simulink model "k1vissr3ta"  (Simulink 8.6)
settings: Solver=VariableStepAuto  StartTime=0.0  StopTime=10.0  RelTol=1e-3
libraries: cdsFilt x4, cdsCDO64 x3, cdsIPCx x3, TYPEB_MASTER x3, cdsCDI64 x2, dac x2, cdsAdcx0 x1, cdsParameters x1
settings Model: Creator=controls  LastModifiedBy=controls
settings DataIOCC: SaveFormat=Dataset  SignalLoggingSaveFormat=Dataset
settings OptimizationCC: ExpressionDepthLimit=128
settings DebuggingCC: UnderspecifiedInitializationDetection=Simplified  MergeDetectMultiDrivingBlocksExec=error  SolverPrmCheckMsg=none  FcnCallInpInsideContextMsg=EnableAllAsError  StateNameClashWarn=none
settings HardwareCC: ProdBitPerPointer=64  ProdLargestAtomicFloat=Float  ProdIntDivRoundTo=Zero  ProdEndianess=LittleEndian  ProdWordSize=64  ProdHWDeviceType=Intel->x86-64 (Windows64)
settings GRTTargetCC: GeneratePreprocessorConditionals=Use local settings  CombineOutputUpdateFcns=on  GRTInterface=off
settings ConfigComp: CovModelRefEnable=off

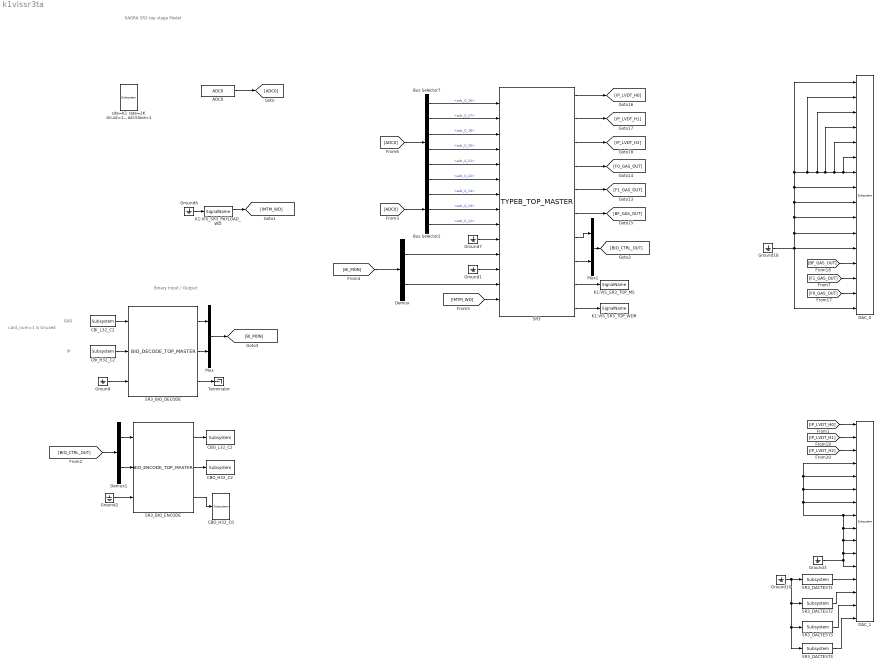
== system k1vissr3ta ==
  note: KAGRA SR3 top stage Model
  note: Binary Input / Output
  note: card_num=1 is Unused
  note: GAS
  note: IP
  ADC0 : cdsAdcx0/ADC0  Tag=cdsAdc  Description=|
      | type-GSC_16AI64SSA
      | card_num=0
      settings: AttributesFormatString=%<Description>\n%<Tag>
  Bus Selector2 : BusSelector  Description=ADC Selector  OutputSignals=adc_0_14,adc_0_13,adc_0_12
      settings: AttributesFormatString=%<Description>
  Bus Selector7 : BusSelector  Description=ADC Selector  OutputSignals=adc_0_16,adc_0_17,adc_0_18,adc_0_20,adc_0_21,adc_0_22
      settings: AttributesFormatString=%<Description>
  CBI_H32_C2 : cdsCDI64/Subsystem  Tag=cdsCDI64  Description=card_num=5
      settings: AttributesFormatString=%<Tag>\n%<Description>
  CBI_L32_C2 : cdsCDI64/Subsystem  Tag=cdsCDI64  Description=card_num=4
      settings: AttributesFormatString=%<Tag>\n%<Description>
  CBO_H32_C0 : cdsCDO64/Subsystem  Tag=cdsCDO64  Description=card_num=1
      settings: AttributesFormatString=%<Tag>\n%<Description>
  CBO_H32_C2 : cdsCDO64/Subsystem  Tag=cdsCDO64  Description=card_num=5
      settings: AttributesFormatString=%<Tag>\n%<Description>
  CBO_L32_C2 : cdsCDO64/Subsystem  Tag=cdsCDO64  Description=card_num=4
      settings: AttributesFormatString=%<Tag>\n%<Description>
  DAC_0 : dac/Subsystem  Description=|
      | type=GSC_16AO16,
      | card_num=0
      settings: AttributesFormatString=%<Description>
  DAC_1 : dac/Subsystem  Description=|
      | type=GSC_16AO16,
      | card_num=1
      settings: AttributesFormatString=%<Description>
  Demux : Demux  Outputs=2
  Demux1 : Demux  Outputs=2
  Ground{,1..3,6..7,10,18} (8 alike) : Ground
  K1:VIS_SR3_PAYLOAD_WD : cdsIPCx/SignalName  Tag=cdsIPCx_SHMEM  Description=Inter-Process Communication via Shared memory.
      settings: AttributesFormatString=%<Tag>
  K1:VIS_SR3_TOP_MS : cdsIPCx/SignalName  Tag=cdsIPCx_SHMEM  Description=Inter-Process Communication via Shared memory.
      settings: AttributesFormatString=%<Tag>
  K1:VIS_SR3_TOP_WDR : cdsIPCx/SignalName  Tag=cdsIPCx_SHMEM  Description=Inter-Process Communication via Shared memory.
      settings: AttributesFormatString=%<Tag>
  Mux : Mux  Inputs=2
  Mux1 : Mux  Inputs=2
  SR3 : TYPEB_MASTER/TYPEB_TOP_MASTER
  SR3_BIO_DECODE : TYPEB_MASTER/BIO_DECODE_TOP_MASTER
  SR3_BIO_ENCODE : TYPEB_MASTER/BIO_ENCODE_TOP_MASTER
  SR3_DACTEST1 : cdsFilt/Subsystem  Tag=cdsFilt  Description=|
      | Purpose:                                                                                                                                                                                                                                  
      | Standard CDS IIR filter module.                                                                                                                                                                                                           
      |                                                                                                                                                                                                                                           
      | Operation:                                                                                                                                                                                                                                
      | Consists of 10 second order section IIR filters, plus a ramped gain stage. In FE code, also provides pre-defined test points and excitation channel inputs. The filter coefficients are defined in the LIGO system using the 'foton' tool.
      |                                                                                                                                                                                                                                           
      | Usage:                                                                                                                                                                                                                                    
      | Name the part with the desired filter module name.
      settings: AttributesFormatString=%<Tag>
  SR3_DACTEST2 : cdsFilt/Subsystem  Tag=cdsFilt  Description=|
      | Purpose:                                                                                                                                                                                                                                  
      | Standard CDS IIR filter module.                                                                                                                                                                                                           
      |                                                                                                                                                                                                                                           
      | Operation:                                                                                                                                                                                                                                
      | Consists of 10 second order section IIR filters, plus a ramped gain stage. In FE code, also provides pre-defined test points and excitation channel inputs. The filter coefficients are defined in the LIGO system using the 'foton' tool.
      |                                                                                                                                                                                                                                           
      | Usage:                                                                                                                                                                                                                                    
      | Name the part with the desired filter module name.
      settings: AttributesFormatString=%<Tag>
  SR3_DACTEST3 : cdsFilt/Subsystem  Tag=cdsFilt  Description=|
      | Purpose:                                                                                                                                                                                                                                  
      | Standard CDS IIR filter module.                                                                                                                                                                                                           
      |                                                                                                                                                                                                                                           
      | Operation:                                                                                                                                                                                                                                
      | Consists of 10 second order section IIR filters, plus a ramped gain stage. In FE code, also provides pre-defined test points and excitation channel inputs. The filter coefficients are defined in the LIGO system using the 'foton' tool.
      |                                                                                                                                                                                                                                           
      | Usage:                                                                                                                                                                                                                                    
      | Name the part with the desired filter module name.
      settings: AttributesFormatString=%<Tag>
  SR3_DACTEST4 : cdsFilt/Subsystem  Tag=cdsFilt  Description=|
      | Purpose:                                                                                                                                                                                                                                  
      | Standard CDS IIR filter module.                                                                                                                                                                                                           
      |                                                                                                                                                                                                                                           
      | Operation:                                                                                                                                                                                                                                
      | Consists of 10 second order section IIR filters, plus a ramped gain stage. In FE code, also provides pre-defined test points and excitation channel inputs. The filter coefficients are defined in the LIGO system using the 'foton' tool.
      |                                                                                                                                                                                                                                           
      | Usage:                                                                                                                                                                                                                                    
      | Name the part with the desired filter module name.
      settings: AttributesFormatString=%<Tag>
  Terminator : Terminator
  site=K1 rate=2K dcuid=1156 host=k1sr3 specific_cpu=6 adcSlave=1 : cdsParameters/Subsystem  Tag=cdsParameters  Description=|
      | Purpose:                                                                                                                                                                                                                                
      | Provide system parameters to the FE code generator to properly configure the generated EPICS names, rep rate of the FE controller, and the Data Acquisition node ID for proper storage of data from this FE controller.                 
      |                                                                                                                                                                                                                                         
      | Useage:                                                                                                                                                                                                                                 
      | The part NAME field is used to identify the FE parameters. It must be of the form:                                                                                                                                                      
      | site=                                                                                                                                                                                                                                   
      | rate=                                                                                                                                                                                                                                   
      | dcuid=                                                                                                                                                                                                                                  
      |                                                                                                                                                                                                                                         
      | Where:                                                                                                                                                                                                                                  
      | site= argument may be H1, H2, L1, M1, G1, either as a single argument or multiple, for example site=H1,H2. These are the only names allowed. These will become the first two characters of all EPICS and signal names (for example G1:).
      |                                                                                                                                                                                                                                         
      | rate= may be 2K, 16K, 32K, or 64K                                                                                                                                                                                                       
      |                                                                                                                                                                                                                                         
      | dcuid= is site specific ie it must be unique at each site.
      settings: AttributesFormatString=%<Tag>
  wires:
  SR3/4 -> [F0_GAS_OUT]
  SR3/5 -> [F1_GAS_OUT]
  SR3/6 -> [BF_GAS_OUT]
  ADC0/1 -> [ADC0]
  [ADC0] -> Bus Selector7/1
  [ADC0] -> Bus Selector2/1
  Bus Selector2/2 -> SR3/8  "<adc_0_13>"
  Bus Selector2/3 -> SR3/9  "<adc_0_12>"
  Bus Selector7/1 -> SR3/1  "<adc_0_16>"
  Bus Selector7/2 -> SR3/2  "<adc_0_17>"
  Bus Selector7/3 -> SR3/3  "<adc_0_18>"
  Bus Selector7/4 -> SR3/4  "<adc_0_20>"
  Bus Selector7/5 -> SR3/5  "<adc_0_21>"
  Bus Selector7/6 -> SR3/6  "<adc_0_22>"
  Ground7/1 -> SR3/10
  Demux/1 -> SR3/11
  [BI_MON] -> Demux/1
  Demux/2 -> SR3/13
  Ground1/1 -> SR3/12
  Mux1/1 -> [BIO_CTRL_OUT]
  SR3/7 -> Mux1/1
  [F1_GAS_OUT] -> DAC_0/14
  [F0_GAS_OUT] -> DAC_0/15
  [BF_GAS_OUT] -> DAC_0/13
  SR3/2 -> [IP_LVDT_H1]
  SR3/1 -> [IP_LVDT_H0]
  SR3/3 -> [IP_LVDT_H2]
  [IP_LVDT_H0] -> DAC_1/1
  [IP_LVDT_H1] -> DAC_1/2
  [IP_LVDT_H2] -> DAC_1/3
  Bus Selector2/1 -> SR3/7  "<adc_0_14>"
  Ground18/1 -> DAC_0/11, DAC_0/10, DAC_0/9, DAC_0/1, DAC_0/2, DAC_0/3, DAC_0/4, DAC_0/5, DAC_0/6, DAC_0/7, DAC_0/8, DAC_0/16, DAC_0/12
  Ground3/1 -> DAC_1/12, DAC_1/7, DAC_1/6, DAC_1/5, DAC_1/4, DAC_1/8, DAC_1/9, DAC_1/10, DAC_1/11
  SR3_DACTEST3/1 -> DAC_1/15
  SR3_DACTEST4/1 -> DAC_1/16
  SR3_DACTEST2/1 -> DAC_1/14
  SR3_DACTEST1/1 -> DAC_1/13
  Ground10/1 -> SR3_DACTEST4/1, SR3_DACTEST3/1, SR3_DACTEST2/1, SR3_DACTEST1/1
  SR3/8 -> Mux1/2
  Ground6/1 -> K1:VIS_SR3_PAYLOAD_WD/1
  K1:VIS_SR3_PAYLOAD_WD/1 -> [IMTM_WD]
  [IMTM_WD] -> SR3/14
  SR3/9 -> K1:VIS_SR3_TOP_MS/1
  SR3/10 -> K1:VIS_SR3_TOP_WDR/1
  SR3_BIO_ENCODE/1 -> CBO_L32_C2/1
  CBI_L32_C2/1 -> SR3_BIO_DECODE/1
  SR3_BIO_DECODE/1 -> Mux/1
  SR3_BIO_DECODE/2 -> Mux/2
  Mux/1 -> [BI_MON]
  [BIO_CTRL_OUT] -> Demux1/1
  CBI_H32_C2/1 -> SR3_BIO_DECODE/2
  SR3_BIO_ENCODE/2 -> CBO_H32_C2/1
  Demux1/2 -> SR3_BIO_ENCODE/2
  Ground/1 -> SR3_BIO_DECODE/3
  SR3_BIO_DECODE/3 -> Terminator/1
  Demux1/1 -> SR3_BIO_ENCODE/1
  SR3_BIO_ENCODE/3 -> CBO_H32_C0/1
  Ground2/1 -> SR3_BIO_ENCODE/3
